simulink model "cellcounting"  (Simulink 9.1)
settings: Solver=FixedStepDiscrete  StartTime=0.0  StopTime=inf  RelTol=1e-3  EnableMultiTasking=on
model workspace: external: MATLAB Code (data not in the file)
undefined symbols (not defined in the file or in its folder): strel
libraries: visiontextngfix x3, visionmorphops x2, visionstatistics x1, simulink x1, visionsinks x1, dspvision x1, visionconversions x1
settings Model: FPTRunName=Active  Creator=The MathWorks Inc.  LastModifiedBy=Master  ExtModeAutoUpdateStatusClock=off
settings DataIOCC: LimitDataPoints=on  SignalLoggingSaveFormat=ModelDataLogs  SaveOutput=off  SignalLogging=off  SaveTime=off
settings OptimizationCC: DefaultParameterBehavior=Inlined  EnhancedBackFolding=on  PassReuseOutputArgsAs=Individual arguments  ExpressionDepthLimit=2147483647  InitFltsAndDblsToZero=on  LifeSpan=auto  BufferReusableBoundary=off  OptimizeBlockOrder=speed  DifferentSizesBufferReuse=on  OptimizationCustomize=off
settings DebuggingCC: SignalResolutionControl=TryResolveAllWithWarning  SolverPrmCheckMsg=warning  MultiTaskDSMMsg=warning  MultiTaskCondExecSysMsg=none  ParameterTunabilityLossMsg=error  FcnCallInpInsideContextMsg=warning  BusObjectLabelMismatch=none  StateNameClashWarn=warning
settings HardwareCC: TargetBitPerPointer=64  TargetBitPerSizeT=64  TargetBitPerPtrDiffT=64  TargetLongLongMode=on  TargetIntDivRoundTo=Zero  TargetEndianess=LittleEndian  TargetWordSize=64  TargetHWDeviceType=Generic->MATLAB Host Computer  ProdEqTarget=off
settings SFSimCC: MATLABDynamicMemAlloc=off
settings RTWCC: SystemTargetFile=ert.tlc  TemplateMakefile=ert_default_tmf  Description=Embedded Coder  GenerateReport=on  IncludeHyperlinkInReport=on  LaunchReport=on  GenerateTraceInfo=on  GenerateTraceReport=on  GenerateTraceReportSl=on  GenerateTraceReportSf=on  GenerateTraceReportEml=on
settings CodeAppCC: ForceParamTrailComments=on  IgnoreCustomStorageClasses=off  OperatorAnnotations=on  SimulinkDataObjDesc=on  SFDataObjDesc=on  MATLABFcnDesc=on  InsertBlockDesc=on  MATLABSourceComments=on  ReqsInCode=on
settings ERTTargetCC: GenerateSampleERTMain=on  SupportVariableSizeSignals=on  InlinedParameterPlacement=NonHierarchical  ERTCustomFileTemplate=example_file_process.tlc

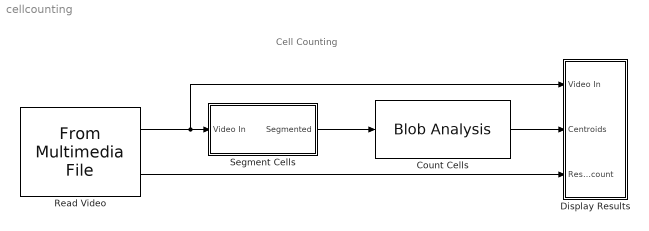
== system cellcounting ==
  note: Cell Counting
  Count Cells : visionstatistics/Blob Analysis  Tag=vipblks_row_conv  area=off  centroid=on  bBox=off  majorAxis=off  minorAxis=off  angle=off  eccentricity=off  equivDiameterSq=off  extent=off  perimeter=off  maxBlobs=1500  warnIfNumBlobsExceeded=on  isCount=off  useMinArea=on  minArea=7  useMaxArea=on  maxArea=300  excludeBorderBlob=off  outDT=single  isOutVarDim=on  isFill=on  fillValues=-10  conn=8  isLabel=off  outputMode=Binary point scaling  outputWordLength=32  outputFracLength=0  firstCoeffMode=Binary point scaling  firstCoeffWordLength=16  firstCoeffFracLength=14  secondCoeffMode=Binary point scaling  secondCoeffWordLength=32  secondCoeffFracLength=16  accumMode=Binary point scaling  accumWordLength=32  accumFracLength=0  prodOutputMode=Binary point scaling  prodOutputWordLength=32  prodOutputFracLength=16  roundingMode=Floor  overflowMode=off
      settings: SourceProductName=Computer Vision System Toolbox
  Display Results : Subsystem
  Read Video : dspvision/From Multimedia File  inputFilename=ecolicells.avi  loop=on  numPlays=inf  outputStreams=Video only  videoDataType=single  audioDataType=int16  inheritSampleTime=off  userDefinedSampleTime=1/30  noAudioOutput=off  isIntensityVideo=off  fourcc=Intensity  colorVideoFormat=Separate color signals  outputEOF=on  dataOrg=Column-major  audioFrameSize=1024  computeAudioFrameSize=off  outSamplingMode=Frame based
      settings: SourceProductBaseCode=VP
  Segment Cells : Subsystem
  wires:
  Segment Cells/1(Segmented) -> Count Cells/1
  Read Video/2 -> Display Results/3(Reset count)
  Count Cells/1 -> Display Results/2(Centroids)
  Read Video/1 -> Segment Cells/1(Video In), Display Results/1(Video In)

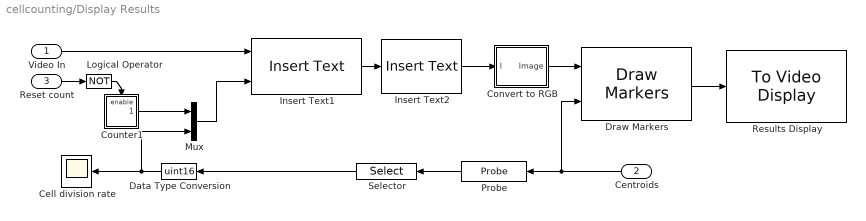
== system cellcounting/Display Results ==
  Video In : Inport
  Centroids : Inport  Port=2
  Reset count : Inport  Port=3
  Cell division rate : Scope
  Convert to RGB : Subsystem
  Counter1 : Subsystem  TreatAsAtomicUnit=on
  Data Type Conversion : DataTypeConversion  OutDataTypeStr=uint16
  Draw Markers : visiontextngfix/Draw Markers  shape=Star  size=2  fill=off  fillClrSource=Specify via dialog  display=User-specified value  intensity=155  color=[1 0 0]  opacity=0  viewport=Entire image  antialiasing=off  inType=Obsolete  imagePorts=One multidimensional signal  prodOutputMode=Binary point scaling  prodOutputWordLength=32  prodOutputFracLength=14  memoryMode=Specify word length  memoryWordLength=16  memoryFracLength=15  roundingMode=Floor  overflowMode=off
      settings: SourceProductName=Computer Vision System Toolbox  SourceProductBaseCode=VP
  Insert Text1 : visiontextngfix/Insert Text  inputType=Obsolete  theText='Frame %d, Count %d'  getTextLocFrom=Specify via dialog  textLoc=[10 11]  getTextColorFrom=Specify via dialog  textColor=1  getTextIntensityFrom=Specify via dialog  textIntensity=1  getTextOpacityFrom=Specify via dialog  textOpacity=1.0  dummyVar2=0  dummyVar3=0  dummyVar4=0  imagePorts=One multidimensional signal  isInputTransposed=off  fontFace=LucidaTypewriterRegular  dummyVar1=0  blockFontSize=16  antiAliased=on
      settings: SourceProductName=Computer Vision System Toolbox  SourceProductBaseCode=VP
  Insert Text2 : visiontextngfix/Insert Text  inputType=Obsolete  theText='Data set courtesy of Jonathan Young and Michael Elowitz, California Institute of Technology'  getTextLocFrom=Specify via dialog  textLoc=[1 417]  getTextColorFrom=Specify via dialog  textColor=1  getTextIntensityFrom=Specify via dialog  textIntensity=1  getTextOpacityFrom=Specify via dialog  textOpacity=1.0  dummyVar2=0  dummyVar3=0  dummyVar4=0  imagePorts=One multidimensional signal  isInputTransposed=off  fontFace=LucidaSansRegular  dummyVar1=0  blockFontSize=12  antiAliased=on
      settings: SourceProductName=Computer Vision System Toolbox  SourceProductBaseCode=VP
  Logical Operator : Logic  Operator=NOT  AllPortsSameDT=off  OutDataTypeStr=boolean
  Mux : Mux  Inputs=2
  Probe : Probe  ProbeWidth=off  ProbeSampleTime=off  ProbeComplexSignal=off  ProbeSignalDimensions=on  ProbeWidthDataType=uint8
  Results Display : visionsinks/To Video Display  windowSizeMode=True size (1:1)  openAtMdlStart=on  fullScreen=off  videoWindowX=115  videoWindowY=153  saveWindowSize=off  videoWindowWidth=528  videoWindowHeight=432  inputColorFormat=RGB  inputType=Obsolete  imagePorts=One multidimensional signal  OutputDevice=On-screen video monitor  dataOrg=Column-major  isWindowOpen=off
      settings: SourceProductName=Computer Vision System Toolbox
  Selector : Selector  NumberOfDimensions=2  InputPortWidth=3  IndexOptions=Index vector (dialog),Index vector (dialog)  Indices=1,1  OutputSizes=99,1
  wires:
  Video In/1 -> Insert Text1/1
  Mux/1 -> Insert Text1/2
  Insert Text1/1 -> Insert Text2/1
  Draw Markers/1 -> Results Display/1
  Centroids/1 -> Draw Markers/2, Probe/1
  Insert Text2/1 -> Convert to RGB/1(I)
  Convert to RGB/1(Image) -> Draw Markers/1
  Probe/1 -> Selector/1
  Selector/1 -> Data Type Conversion/1
  Data Type Conversion/1 -> Mux/2, Cell division rate/1
  Logical Operator/1 -> Counter1/Enable
  Counter1/1(Out1) -> Mux/1
  Reset count/1 -> Logical Operator/1

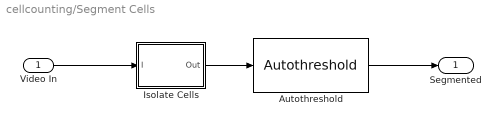
== system cellcounting/Segment Cells ==
  Video In : Inport
  Autothreshold : visionconversions/Autothreshold  operator=<=  threshOut=off  effMetricOut=off  userDefinedRange=off  umin=0  umax=1  outOfRngOpt=Warn and saturate  scaleThreshold=on  scaleFactor=single(0.8)  P1Mode=Specify word length  P1WordLength=32  P1FracLength=30  P2Mode=Specify word length  P2WordLength=32  P2FracLength=22  P3Mode=Specify word length  P3WordLength=32  P3FracLength=14  P4Mode=Binary point scaling  P4WordLength=32  P4FracLength=15  Q1Mode=Specify word length  Q1WordLength=32  Q1FracLength=16  EMMode=Specify word length  EMWordLength=16  EMFracLength=14  roundingMode=Floor  overflowMode=off
      settings: SourceProductName=Computer Vision System Toolbox  SourceProductBaseCode=VP
  Isolate Cells : Subsystem
  Segmented : Outport
  wires:
  Video In/1 -> Isolate Cells/1(I)
  Isolate Cells/1(Out) -> Autothreshold/1
  Autothreshold/1 -> Segmented/1

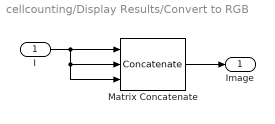
== system cellcounting/Display Results/Convert to RGB ==
  I : Inport
  Matrix Concatenate : Concatenate  NumInputs=3  Mode=Multidimensional array  ConcatenateDimension=3
  Image : Outport
  wires:
  I/1 -> Matrix Concatenate/1, Matrix Concatenate/2, Matrix Concatenate/3
  Matrix Concatenate/1 -> Image/1

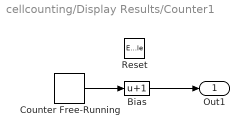
== system cellcounting/Display Results/Counter1 ==
  Reset : EnablePort  StatesWhenEnabling=reset
  Bias : Bias  Bias=1
  Counter Free-Running : simulink/Sources/Counter Free-Running  NumBits=16  tsamp=1/30
  Out1 : Outport
  wires:
  Counter Free-Running/1 -> Bias/1
  Bias/1 -> Out1/1

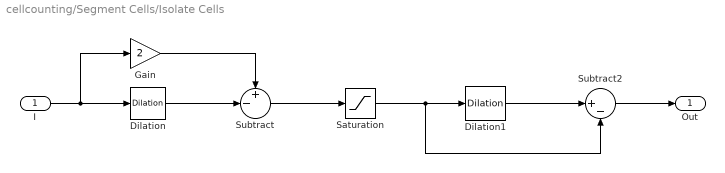
== system cellcounting/Segment Cells/Isolate Cells ==
  I : Inport
  Dilation : visionmorphops/Dilation  nhoodsrc=Specify via dialog  strel=strel('square',7)
      settings: SourceProductName=Computer Vision System Toolbox  SourceProductBaseCode=VP
  Dilation1 : visionmorphops/Dilation  nhoodsrc=Specify via dialog  strel=strel('square',7)
      settings: SourceProductName=Computer Vision System Toolbox  SourceProductBaseCode=VP
  Gain : Gain  Gain=2
  Saturation : Saturate  UpperLimit=1  LowerLimit=0
  Subtract : Sum  Inputs=+-|  SaturateOnIntegerOverflow=on
  Subtract2 : Sum  Inputs=|+-  SaturateOnIntegerOverflow=on
  Out : Outport
  wires:
  Subtract2/1 -> Out/1
  I/1 -> Dilation/1, Gain/1
  Subtract/1 -> Saturation/1
  Dilation1/1 -> Subtract2/1
  Saturation/1 -> Dilation1/1, Subtract2/2
  Dilation/1 -> Subtract/2
  Gain/1 -> Subtract/1
